simulink model "Simulation_Parallel"  (R2025b)
settings: Solver=ode23tb  StartTime=0.0  StopTime=30000  RelTol=1e-4  AbsTol=1e-4  EnableMultiTasking=on
PreLoadFcn:
  | addpath(genpath(fileparts(bdroot)));
  | disp('Model loaded: Added subfolders to path.');
InitFcn:
  | %if exist('optiver') > 1
  | %    % OptiToolBox is installed
  | %   disp('OptiToolBox is installed');
  | %else
  | %    cd ../OptiToolbox;
  | %    unzip OPTIToolbox.zip;
  |  %   run opti_Install;
  | %    cd ../../../../Loadsharing;
  | % end
  | 
  | clear all
  | %Mpcparam
  | X_init_1;
values from neighbouring files (symbols this model uses):
  X1 = [97725.7043981493 ... (first row only)    [X_init_parallel.m]
  X2 = X1    [X_init_parallel.m]
libraries: simulink x4, slpidlib x3
settings Model: SimulationMode=accelerator  Creator=chancor1  LastModifiedBy=ld719
settings SolverCC: AlgebraicLoopSolver=TrustRegion
settings DataIOCC: LimitDataPoints=on  SaveFinalState=on  SaveFormat=Array  SignalLoggingSaveFormat=ModelDataLogs  ReturnWorkspaceOutputs=off
settings OptimizationCC: ExpressionDepthLimit=2147483647.0  LifeSpan=inf
settings DebuggingCC: UnderspecifiedInitializationDetection=Classic  MergeDetectMultiDrivingBlocksExec=none  SolverPrmCheckMsg=warning  FcnCallInpInsideContextMsg=warning  UnconnectedInputMsg=warning  UnconnectedOutputMsg=warning  UnconnectedLineMsg=warning  StateNameClashWarn=warning  SFUnexpectedBacktrackingDiag=warning  SFNoUnconditionalDefaultTransitionDiag=warning  SFExecutionAtInitializationDiag=none  ArithmeticOperatorsInVariantConditions=warning
settings HardwareCC: ProdBitPerPointer=32.0  ProdBitPerSizeT=32.0  ProdBitPerPtrDiffT=32.0  ProdLargestAtomicFloat=None  ProdIntDivRoundTo=Undefined  ProdEndianess=Unspecified  ProdWordSize=32.0  ProdHWDeviceType=32-bit Generic
settings ModelReferenceCC: EnableRefExpFcnMdlSchedulingChecks=on  PropagateSignalLabelsOutOfModel=off
settings SFSimCC: SimUseLocalCustomCode=off  CustomCodeUndefinedFunction=UseInterfaceOnly
settings RTWCC: RTWUseLocalCustomCode=off  GPUComputeCapability=3.5
settings CodeAppCC: StateflowObjectComments=on
settings GRTTargetCC: TargetLangStandard=C89/C90 (ANSI)  CombineOutputUpdateFcns=off  GRTInterface=on
settings ConfigComp: CovMetricSettings=dw  CovSaveCumulativeToWorkspaceVar=on  CovSaveSingleToWorkspaceVar=on  CovExternalEMLEnable=off  CovSFcnEnable=off

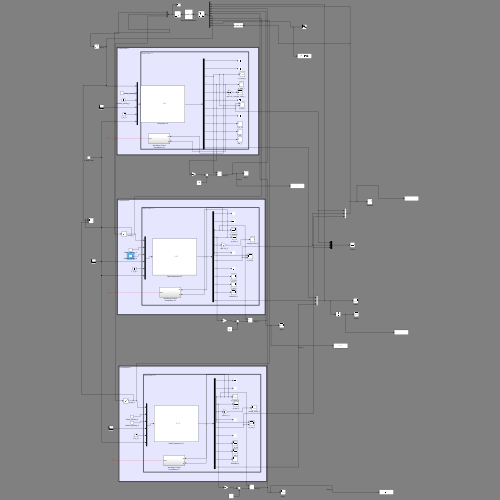
[thumbnail: Simulink's stored preview of the top-level diagram]
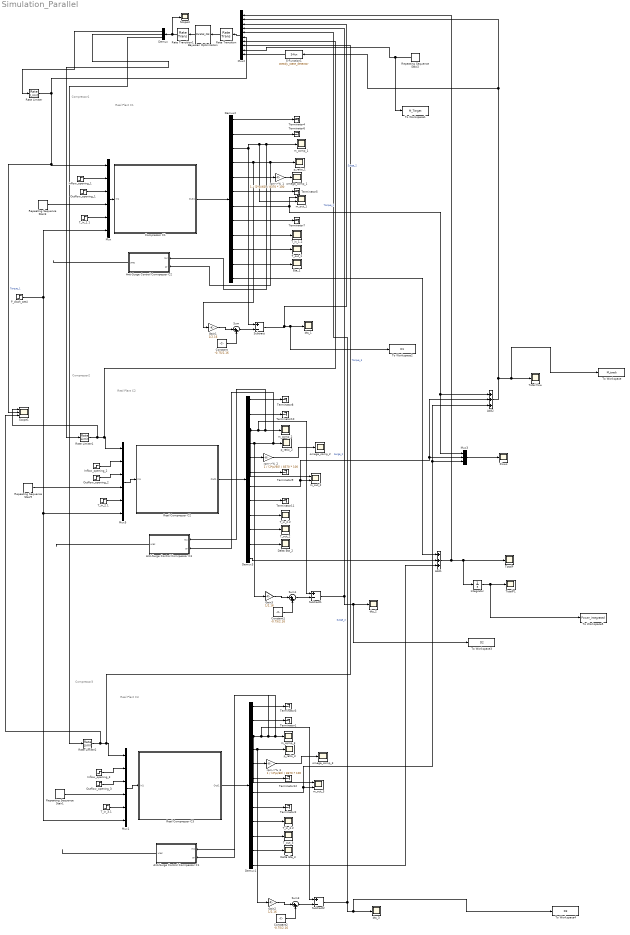
== system Simulation_Parallel ==
  note: Real Plant C2
  note: Real Plant C1
  note: Compressor2
  note: Compressor1
  note: Compressor3
  note: Real Plant C3
  Add1 : Sum  Inputs=+++
  Add2 : Sum  Inputs=+++
  Anti-Surge Control Comrpessor C1 : Subsystem
  Anti-Surge Control Comrpessor C2 : Subsystem
  Anti-Surge Control Comrpessor C3 : Subsystem
  Bayesian Optimization : S-Function  FunctionName=Parallel_CEI  SFunctionDeploymentMode=off  EnableBusSupport=off
  Compressor C1 : Subsystem
      mask Display: image(imread('comp_plant.jpg'))
  Constant : Constant  Value=-0.75/2.16
  Constant1 : Constant  Value=-0.75/2.16
  Constant2 : Constant  Value=-0.75/2.16
  Delta Eta_2 : Scope
      settings: TimeSpan=400  ActiveDisplayYMinimum=0.71048158275738349  ActiveDisplayYMaximum=0.91746637910547824  DataLoggingVariableName=m_rec16  DataLoggingSaveFormat=Array
  Delta Eta_3 : Scope
      settings: TimeSpan=400  ActiveDisplayYMinimum=0.57039067870256488  ActiveDisplayYMaximum=0.76995457969756409  DataLoggingVariableName=m_rec4  DataLoggingSaveFormat=Array
  Demux : Demux  Outputs=3
  Demux1 : Demux  Outputs=12
  Demux2 : Demux  Outputs=12
  Demux3 : Demux  Outputs=12
  Eta_1 : Scope
      settings: TimeSpan=500  ActiveDisplayYMinimum=0.2397543776883454  ActiveDisplayYMaximum=0.63682038343790071  DataLoggingVariableName=m_rec16  DataLoggingSaveFormat=Array
  Flows : Scope
      settings: TimeSpan=500  ActiveDisplayYMinimum=0.36309368835206474  ActiveDisplayYMaximum=0.74236027172168861  DataLoggingVariableName=Individual_Flows  DataLoggingSaveFormat=Array
  Gain1 : Gain  Gain=1/2.16
  Gain2 : Gain  Gain=1/2.16
  Gain3 : Gain  Gain=1/2.16
  Inflow_opening_1 : Step  Time=25  Before=0.4541  After=0.4541  SampleTime=0
  Inflow_opening_2 : Step  Time=25  Before=0.4541  After=0.4541  SampleTime=0
  Inflow_opening_3 : Step  Time=25  Before=0.4541  After=0.4541  SampleTime=0
  Integrator : Integrator
  Mux : Mux  Inputs=6
  Mux1 : Mux  Inputs=6
  Mux2 : Mux  Inputs=10
  Mux3 : Mux  Inputs=3
  Mux5 : Mux  Inputs=6
  Outflow_opening_1 : Step  Time=30  Before=0.56  After=0.56  SampleTime=0
  Outflow_opening_2 : Step  Time=30  Before=0.56  After=0.56  SampleTime=0
  Outflow_opening_3 : Step  Time=30  Before=0.56  After=0.56  SampleTime=0
  P_disch_set4 : Step  Time=4000  Before=155000  After=155000  SampleTime=0
  Rate Limiter : RateLimiter  RisingSlewLimit=0.1  FallingSlewLimit=-0.1  SampleTimeMode=inherited
  Rate Limiter1 : RateLimiter  RisingSlewLimit=0.1  FallingSlewLimit=-0.1  SampleTimeMode=inherited
  Rate Limiter2 : RateLimiter  RisingSlewLimit=0.1  FallingSlewLimit=-0.1  SampleTimeMode=inherited
  Rate Transition : RateTransition
  Rate Transition1 : RateTransition  InitialCondition=[15;15;15]
  Real Compressor C2 : Subsystem
      mask Display: image(imread('comp_plant.jpg'))
  Real Compressor C3 : Subsystem
      mask Display: image(imread('comp_plant.jpg'))
  Repeating Sequence Stair1 : simulink/Sources/Repeating Sequence Stair  OutValues=[0].'  tsamp=-1  OutMin=[]  OutMax=[]  OutDataTypeStr=double  OutputDataTypeScalingMode=double  OutDataType=fixdt(0,8)  ConRadixGroup=Best Precision: Vector-wise  OutScaling=2^-12
  Repeating Sequence Stair2 : simulink/Sources/Repeating Sequence Stair  OutValues=[2.1 1.8 1.9 1.7 1.6 1.5 ].'  tsamp=5000  OutMin=[]  OutMax=[]  OutDataTypeStr=double  OutputDataTypeScalingMode=double  OutDataType=fixdt(0,8)  ConRadixGroup=Best Precision: Vector-wise  OutScaling=2^-12
  Repeating Sequence Stair3 : simulink/Sources/Repeating Sequence Stair  OutValues=[0].'  tsamp=-1  OutMin=[]  OutMax=[]  OutDataTypeStr=double  OutputDataTypeScalingMode=double  OutDataType=fixdt(0,8)  ConRadixGroup=Best Precision: Vector-wise  OutScaling=2^-12
  Repeating Sequence Stair9 : simulink/Sources/Repeating Sequence Stair  OutValues=[0].'  tsamp=-1  OutMin=[]  OutMax=[]  OutDataTypeStr=double  OutputDataTypeScalingMode=double  OutDataType=fixdt(0,8)  ConRadixGroup=Best Precision: Vector-wise  OutScaling=2^-12
  S-Function1 : S-Function  FunctionName=steady_state_detector  SFunctionDeploymentMode=off  EnableBusSupport=off
  Scope1 : Scope  NumInputPorts=3
      settings: ActiveDisplayYMinimum=7.5235070284689751  ActiveDisplayYMaximum=22.497388107947891  DataLoggingVariableName=ScopeData4
  Scope4 : Scope
      settings: ActiveDisplayYMinimum=9.125  ActiveDisplayYMaximum=27.875
  Subtract : Sum  Inputs=+-
  Subtract1 : Sum  Inputs=+-
  Subtract2 : Sum  Inputs=+-
  Sum : Sum  Inputs=|++
  Sum1 : Sum  Inputs=|++
  Sum3 : Sum  Inputs=|++
  T_in_1.1 : Step  Time=2  Before=273+20  After=273+20  SampleTime=0
  T_in_1.2 : Scope
      settings: ActiveDisplayYMinimum=278.35  ActiveDisplayYMaximum=307.65  DataLoggingVariableName=m_rec1  DataLoggingSaveFormat=Array
  T_in_2.1 : Step  Time=2  Before=273+20  After=273+20  SampleTime=0
  T_in_2.2 : Scope
      settings: ActiveDisplayYMinimum=1.41031E-278  ActiveDisplayYMaximum=8E-262  DataLoggingVariableName=m_rec1  DataLoggingSaveFormat=Array
  T_in_3.1 : Step  Time=2  Before=273+20  After=273+20  SampleTime=0
  T_in_3.2 : Scope
      settings: ActiveDisplayYMinimum=1.41031E-278  ActiveDisplayYMaximum=8E-262  DataLoggingVariableName=m_rec5  DataLoggingSaveFormat=Array
  T_out_1 : Scope
      settings: TimeSpan=100  ActiveDisplayYMinimum=335.8022  ActiveDisplayYMaximum=433.80571  DataLoggingVariableName=m_rec2  DataLoggingSaveFormat=Array
  T_out_2 : Scope
      settings: TimeSpan=100  ActiveDisplayYMinimum=370.79785  ActiveDisplayYMaximum=427.9001  DataLoggingVariableName=m_rec2  DataLoggingSaveFormat=Array
  T_out_3 : Scope
      settings: TimeSpan=100  ActiveDisplayYMinimum=370.79785  ActiveDisplayYMaximum=427.9001  DataLoggingVariableName=m_rec6  DataLoggingSaveFormat=Array
  Terminator{1..12} (12 alike) : Terminator
  To Workspace : ToWorkspace  VariableName=M_track  SaveFormat=Structure With Time  SampleTime=1
  To Workspace1 : ToWorkspace  VariableName=M_Target  SaveFormat=Structure With Time  SampleTime=1
  To Workspace2 : ToWorkspace  VariableName=D1  SaveFormat=Structure With Time  SampleTime=1
  To Workspace3 : ToWorkspace  VariableName=D2  SaveFormat=Structure With Time  SampleTime=1
  To Workspace4 : ToWorkspace  VariableName=D3  SaveFormat=Structure With Time  SampleTime=1
  To Workspace5 : ToWorkspace  VariableName=Power_integrated  SaveFormat=Structure With Time  SampleTime=1
  Total flow : Scope
      settings: TimeSpan=30000  ActiveDisplayYMinimum=1.2722600118252789  ActiveDisplayYMaximum=2.1997897754564577  DataLoggingVariableName=Individual_Flows1  DataLoggingSaveFormat=Array
  TotalP : Scope
      settings: ActiveDisplayYMinimum=126510.3736500807  ActiveDisplayYMaximum=352840.8765047628  DataLoggingVariableName=TotalP  DataLoggingSaveFormat=Array
  TotalP1 : Scope
      settings: ActiveDisplayYMinimum=6.1318455800186586E+9  ActiveDisplayYMaximum=6.1318558553426237E+9  DataLoggingVariableName=TotalE  DataLoggingSaveFormat=Array
  dts_1 : Scope
      settings: TimeSpan=500  ActiveDisplayYMinimum=0.005652196127564145  ActiveDisplayYMaximum=0.23223162651311186  DataLoggingVariableName=m_rec  DataLoggingSaveFormat=Array
  dts_2 : Scope
      settings: TimeSpan=500  ActiveDisplayYMinimum=-0.014136511221945931  ActiveDisplayYMaximum=0.23443037177416717  DataLoggingVariableName=m_rec3  DataLoggingSaveFormat=Array
  dts_3 : Scope
      settings: TimeSpan=500  ActiveDisplayYMinimum=-0.030750707158997012  ActiveDisplayYMaximum=0.23627639354495333  DataLoggingVariableName=m_rec7  DataLoggingSaveFormat=Array
  m_comp_1 : Scope
      settings: TimeSpan=100  ActiveDisplayYMinimum=60.15587  ActiveDisplayYMaximum=126.64848  DataLoggingVariableName=m_comp_C1  DataLoggingSaveFormat=Array
  m_comp_2 : Scope
      settings: TimeSpan=100  ActiveDisplayYMinimum=38.57766  ActiveDisplayYMaximum=113.2372  DataLoggingVariableName=m_comp_C2  DataLoggingSaveFormat=Array
  m_comp_3 : Scope
      settings: TimeSpan=100  ActiveDisplayYMinimum=38.57766  ActiveDisplayYMaximum=113.2372  DataLoggingVariableName=m_comp_C  DataLoggingSaveFormat=Array
  m_out_1 : Scope  NumInputPorts=2
      settings: ActiveDisplayYMinimum=0.47698487803056794  ActiveDisplayYMaximum=0.61709914190973469  DataLoggingVariableName=ScopeData3
  m_out_2 : Scope  NumInputPorts=2
      settings: ActiveDisplayYMinimum=61.12166  ActiveDisplayYMaximum=116.4647  DataLoggingVariableName=ScopeData2
  m_out_3 : Scope  NumInputPorts=2
      settings: ActiveDisplayYMinimum=-1  ActiveDisplayYMaximum=1
  omega_comp_1 : Scope
      settings: TimeSpan=10  ActiveDisplayYMinimum=55.77307  ActiveDisplayYMaximum=77.75846  DataLoggingVariableName=ScopeData5
  omega_comp_2 : Scope
      settings: TimeSpan=10  ActiveDisplayYMinimum=20000  ActiveDisplayYMaximum=120000  DataLoggingVariableName=ScopeData5
  omega_comp_3 : Scope
      settings: TimeSpan=10  ActiveDisplayYMinimum=20000  ActiveDisplayYMaximum=120000  DataLoggingVariableName=ScopeData6
  p_ratio_1 : Scope
      settings: TimeSpan=20  ActiveDisplayYMinimum=1.533809798369548  ActiveDisplayYMaximum=1.8504440162741049  DataLoggingVariableName=p_ratio_C1  DataLoggingSaveFormat=Array
  p_ratio_2 : Scope
      settings: TimeSpan=20  ActiveDisplayYMinimum=-1  ActiveDisplayYMaximum=1  DataLoggingVariableName=p_ratio_C2  DataLoggingSaveFormat=Array
  p_ratio_3 : Scope
      settings: TimeSpan=20  ActiveDisplayYMinimum=-1  ActiveDisplayYMaximum=1  DataLoggingVariableName=p_ratio_C  DataLoggingSaveFormat=Array
  rpm->%_1 : Gain  Gain=1 / (2*pi/60) / 8370 * 100
  rpm->%_2 : Gain  Gain=1 / (2*pi/60) / 8370 * 100
  rpm->%_3 : Gain  Gain=1 / (2*pi/60) / 8370 * 100
  wires:
  Demux2/7 -> m_out_1/1, Mux3/1, Add2/1
  Demux3/7 -> Add2/2, Mux3/2, m_out_2/2
  Mux3/1 -> Flows/1
  Demux3/12 -> Add1/2
  Demux2/12 -> Add1/1
  Demux2/11 -> Eta_1/1
  Demux2/4 -> Gain1/1, Anti-Surge Control Comrpessor C2/2(pr), p_ratio_1/1
  Demux2/3 -> Anti-Surge Control Comrpessor C2/1(mc), m_comp_1/1, m_out_1/2, Subtract/1
  T_in_1.1/1 -> Mux/5
  Outflow_opening_1/1 -> Mux/3
  Inflow_opening_1/1 -> Mux/2
  Demux3/11 -> Delta Eta_2/1
  Demux3/4 -> Anti-Surge Control Comrpessor C3/2(pr), p_ratio_2/1, Gain3/1
  Demux3/3 -> Subtract1/1, Anti-Surge Control Comrpessor C3/1(mc), m_comp_2/1, m_out_2/1
  T_in_2.1/1 -> Mux5/5
  Outflow_opening_2/1 -> Mux5/3
  Inflow_opening_2/1 -> Mux5/2
  P_disch_set4/1 -> Mux1/6, Mux5/6, Mux/6
  Compressor C1/1(Out1) -> Demux2/1
  Mux/1 -> Compressor C1/1(In1)
  rpm->%_1/1 -> omega_comp_1/1
  Demux2/10 -> T_out_1/1
  Demux2/9 -> T_in_1.2/1
  Demux2/8 -> Terminator7/1
  Demux2/2 -> Terminator6/1
  Demux2/1 -> Terminator4/1
  Demux2/6 -> Terminator5/1
  Demux2/5 -> rpm->%_1/1
  Real Compressor C2/1(Out1) -> Demux3/1
  Mux5/1 -> Real Compressor C2/1(In1)
  rpm->%_2/1 -> omega_comp_2/1
  Demux3/10 -> T_out_2/1
  Demux3/9 -> T_in_2.2/1
  Demux3/8 -> Terminator11/1
  Demux3/2 -> Terminator10/1
  Demux3/1 -> Terminator8/1
  Demux3/6 -> Terminator9/1
  Demux3/5 -> rpm->%_2/1
  Sum/1 -> Subtract/2
  Gain1/1 -> Sum/1
  Constant/1 -> Sum/2
  Gain3/1 -> Sum1/1
  Constant1/1 -> Sum1/2
  Sum1/1 -> Subtract1/2
  Rate Transition1/1 -> Scope4/1, Demux/1
  Rate Transition/1 -> Bayesian Optimization/1
  Mux2/1 -> Rate Transition/1
  Bayesian Optimization/1 -> Rate Transition1/1
  Add1/1 -> TotalP/1, Integrator/1, Mux2/1
  Demux/1 -> Rate Limiter/1
  Rate Limiter/1 -> Mux2/6, Scope1/2, Mux/1  "Torque_1"
  Demux/2 -> Rate Limiter1/1
  Rate Limiter1/1 -> Scope1/1, Mux2/7, Mux5/1  "Torque_2"
  S-Function1/1 -> Mux2/10
  Constant2/1 -> Sum3/2
  Demux1/3 -> Subtract2/1, Anti-Surge Control Comrpessor C1/1(mc), Anti-Surge Control Comrpessor C1/2(pr), m_comp_3/1, m_out_3/1
  T_in_3.1/1 -> Mux1/5
  Demux/3 -> Rate Limiter2/1
  rpm->%_3/1 -> omega_comp_3/1
  Demux1/6 -> Terminator12/1
  Outflow_opening_3/1 -> Mux1/3
  Real Compressor C3/1(Out1) -> Demux1/1
  Gain2/1 -> Sum3/1
  Sum3/1 -> Subtract2/2
  Demux1/7 -> Add2/3, Mux3/3, m_out_3/2
  Demux1/9 -> T_in_3.2/1
  Mux1/1 -> Real Compressor C3/1(In1)
  Demux1/8 -> Terminator2/1
  Rate Limiter2/1 -> Scope1/3, Mux2/8, Mux1/1  "Torque_3"
  Demux1/10 -> T_out_3/1
  Demux1/4 -> p_ratio_3/1, Gain2/1
  Demux1/1 -> Terminator3/1
  Inflow_opening_3/1 -> Mux1/2
  Demux1/11 -> Delta Eta_3/1
  Demux1/5 -> rpm->%_3/1
  Demux1/12 -> Add1/3
  Demux1/2 -> Terminator1/1
  Repeating Sequence Stair2/1 -> Mux2/9, To Workspace1/1
  Add2/1 -> S-Function1/1, Mux2/2, To Workspace/1, Total flow/1
  Subtract/1 -> Mux2/3, To Workspace2/1, dts_1/1  "Surge_2"
  Subtract1/1 -> Mux2/4, To Workspace3/1, dts_2/1  "Surge_2"
  Subtract2/1 -> Mux2/5, To Workspace4/1, dts_3/1  "Surge_2"
  Integrator/1 -> To Workspace5/1, TotalP1/1
  Anti-Surge Control Comrpessor C2/1(urec) -> ?
  Anti-Surge Control Comrpessor C3/1(urec) -> ?
  Anti-Surge Control Comrpessor C1/1(urec) -> ?
  Repeating Sequence Stair3/1 -> Mux/4
  Repeating Sequence Stair9/1 -> Mux5/4
  Repeating Sequence Stair1/1 -> Mux1/4

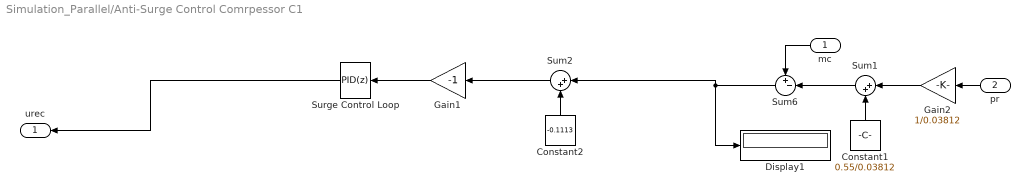
== system Simulation_Parallel/Anti-Surge Control Comrpessor C1 ==
  mc : Inport
  pr : Inport  Port=2
  Constant1 : Constant  Value=0.55/0.03812
  Constant2 : Constant  Value=-0.1113
  Display1 : Display
  Gain1 : Gain  Gain=-1
  Gain2 : Gain  Gain=1/0.03812
  Sum1 : Sum  Inputs=|++
  Sum2 : Sum  Inputs=|++
  Sum6 : Sum  Inputs=+-|
  Surge Control Loop : slpidlib/PID Controller  Controller=PID  Form=Parallel  TimeDomain=Discrete-time  UseExternalTs=off  SampleTime=0.5  IntegratorMethod=Forward Euler  FilterMethod=Forward Euler  ControllerParametersSource=internal  P=0.05  I=0.01  UseKiTs=off  D=0  UseExternalDerivativeSource=off  N=2.82959055969234  UseFilter=on  TunerSelectOption=Transfer Function Based (PID Tuner App)  ZeroCross=off  InitialConditionSource=internal  InitialConditionForIntegrator=0  InitialConditionForFilter=0  DifferentiatorICPrevScaledInput=0  ExternalReset=none  TrackingMode=off  Kt=1  LimitOutput=on  SatLimitsSource=internal  UpperSaturationLimit=1  LowerSaturationLimit=0  LinearizeAsGain=off  AntiWindupMode=back-calculation  Kb=1  LimitIntegrator=off  UpperIntegratorSaturationLimit=inf  LowerIntegratorSaturationLimit=-inf  POutMin=[]  POutMax=[]  IOutMin=[]  IOutMax=[]  DOutMin=[]  DOutMax=[]  NOutMin=[]  NOutMax=[]  SumOutMin=[]  SumOutMax=[]  SaturationOutMin=[]  SaturationOutMax=[]  PParamMin=[]  PParamMax=[]  IParamMin=[]  IParamMax=[]  DParamMin=[]  DParamMax=[]  NParamMin=[]  NParamMax=[]  KbParamMin=[]  KbParamMax=[]  KtParamMin=[]  KtParamMax=[]  KbOutMin=[]  KbOutMax=[]  KtOutMin=[]  KtOutMax=[]  IntegratorOutMin=[]  IntegratorOutMax=[]  FilterOutMin=[]  FilterOutMax=[]  SumI1OutMin=[]  SumI1OutMax=[]  SumI2OutMin=[]  SumI2OutMax=[]  SumI3OutMin=[]  SumI3OutMax=[]  SumI4OutMin=[]  SumI4OutMax=[]  SumDOutMin=[]  SumDOutMax=[]  DifferentiatorOutMin=[]  DifferentiatorOutMax=[]  FilterDiffOutCoefMin=[]  FilterDiffOutCoefMax=[]  ReciprocalOutMin=[]  ReciprocalOutMax=[]  SumDenOutMin=[]  SumDenOutMax=[]  SumNumOutMin=[]  SumNumOutMax=[]  DivideOutMin=[]  DivideOutMax=[]  UdiffTsProdOutMin=[]  UdiffTsProdOutMax=[]  NTsProdOutMin=[]  NTsProdOutMax=[]  UintegralTsProdOutMin=[]  UintegralTsProdOutMax=[]  UngainTsProdOutMin=[]  UngainTsProdOutMax=[]  ClampingZeroOutDataTypeStr=Inherit: Inherit via back propagation  ClampingZeroOutMin=[]  ClampingZeroOutMax=[]  FilterDenConstantOutDataTypeStr=Inherit: Inherit via back propagation  FilterDenConstantOutMin=[]  FilterDenConstantOutMax=[]  PCopyOutDataTypeStr=Inherit: Inherit via back propagation  PCopyOutMin=[]  PCopyOutMax=[]  NCopyOutDataTypeStr=Inherit: Inherit via back propagation  NCopyOutMin=[]  NCopyOutMax=[]  IntegratorContinuousStateAttributes=''  IntegratorStateMustResolveToSignalObject=off  IntegratorRTWStateStorageClass=Auto  FilterContinuousStateAttributes=''  FilterStateMustResolveToSignalObject=off  FilterRTWStateStorageClass=Auto  ParallelPVariant=InternalParameters  IdealPVariant=Disabled  IVariant=InternalParameters  DVariant=InternalParameters  IntegratorVariant=Discrete  SatVariant=Enabled  AWVariant=BackCalculation  PCopyVariant=Disabled  TRVariant=Disabled  FdbkBlocksVariant=Forward  IdealPFdbkVariant=Disabled  SatFdbkVariant=Disabled  DerivativeFilterVariant=ForwardEulerFilter  NVariant=InternalParameters  NCopyVariant=Disabled  FilterICVariant=InternalICsFilter  IntegratorICVariant=InternalICs  ExternalResetVariant=Disabled  TRSumVariant=Passthrough  SumFdbkVariant=Disabled  SumVariant=Sum_PID  TsampFilterVariant=InternalTs  TsampNgainVariant=Passthrough  TsampIntegralVariant=Disabled_SignalSpec  ExternalSaturationOutDataTypeStr=Inherit: Same as second input  DerivativeSourceVariant=ErrorSignal  PreIntVariant=InternalPreInt
  urec : Outport
  wires:
  Gain2/1 -> Sum1/1
  Constant1/1 -> Sum1/2
  Sum1/1 -> Sum6/2
  Sum6/1 -> Sum2/1, Display1/1
  Surge Control Loop/1 -> urec/1
  mc/1 -> Sum6/1
  pr/1 -> Gain2/1
  Gain1/1 -> Surge Control Loop/1
  Sum2/1 -> Gain1/1
  Constant2/1 -> Sum2/2

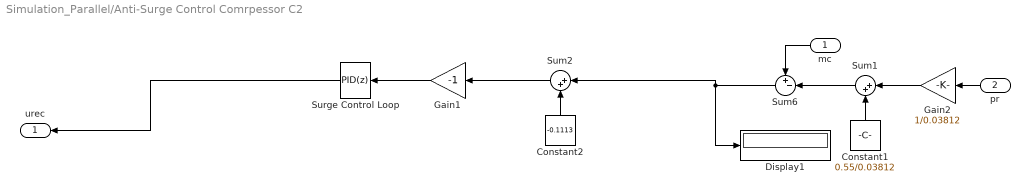
== system Simulation_Parallel/Anti-Surge Control Comrpessor C2 ==
  mc : Inport
  pr : Inport  Port=2
  Constant1 : Constant  Value=0.55/0.03812
  Constant2 : Constant  Value=-0.1113
  Display1 : Display
  Gain1 : Gain  Gain=-1
  Gain2 : Gain  Gain=1/0.03812
  Sum1 : Sum  Inputs=|++
  Sum2 : Sum  Inputs=|++
  Sum6 : Sum  Inputs=+-|
  Surge Control Loop : slpidlib/PID Controller  Controller=PID  Form=Parallel  TimeDomain=Discrete-time  UseExternalTs=off  SampleTime=0.5  IntegratorMethod=Forward Euler  FilterMethod=Forward Euler  ControllerParametersSource=internal  P=0.05  I=0.01  UseKiTs=off  D=0  UseExternalDerivativeSource=off  N=2.82959055969234  UseFilter=on  TunerSelectOption=Transfer Function Based (PID Tuner App)  ZeroCross=off  InitialConditionSource=internal  InitialConditionForIntegrator=0  InitialConditionForFilter=0  DifferentiatorICPrevScaledInput=0  ExternalReset=none  TrackingMode=off  Kt=1  LimitOutput=on  SatLimitsSource=internal  UpperSaturationLimit=1  LowerSaturationLimit=0  LinearizeAsGain=off  AntiWindupMode=back-calculation  Kb=1  LimitIntegrator=off  UpperIntegratorSaturationLimit=inf  LowerIntegratorSaturationLimit=-inf  POutMin=[]  POutMax=[]  IOutMin=[]  IOutMax=[]  DOutMin=[]  DOutMax=[]  NOutMin=[]  NOutMax=[]  SumOutMin=[]  SumOutMax=[]  SaturationOutMin=[]  SaturationOutMax=[]  PParamMin=[]  PParamMax=[]  IParamMin=[]  IParamMax=[]  DParamMin=[]  DParamMax=[]  NParamMin=[]  NParamMax=[]  KbParamMin=[]  KbParamMax=[]  KtParamMin=[]  KtParamMax=[]  KbOutMin=[]  KbOutMax=[]  KtOutMin=[]  KtOutMax=[]  IntegratorOutMin=[]  IntegratorOutMax=[]  FilterOutMin=[]  FilterOutMax=[]  SumI1OutMin=[]  SumI1OutMax=[]  SumI2OutMin=[]  SumI2OutMax=[]  SumI3OutMin=[]  SumI3OutMax=[]  SumI4OutMin=[]  SumI4OutMax=[]  SumDOutMin=[]  SumDOutMax=[]  DifferentiatorOutMin=[]  DifferentiatorOutMax=[]  FilterDiffOutCoefMin=[]  FilterDiffOutCoefMax=[]  ReciprocalOutMin=[]  ReciprocalOutMax=[]  SumDenOutMin=[]  SumDenOutMax=[]  SumNumOutMin=[]  SumNumOutMax=[]  DivideOutMin=[]  DivideOutMax=[]  UdiffTsProdOutMin=[]  UdiffTsProdOutMax=[]  NTsProdOutMin=[]  NTsProdOutMax=[]  UintegralTsProdOutMin=[]  UintegralTsProdOutMax=[]  UngainTsProdOutMin=[]  UngainTsProdOutMax=[]  ClampingZeroOutDataTypeStr=Inherit: Inherit via back propagation  ClampingZeroOutMin=[]  ClampingZeroOutMax=[]  FilterDenConstantOutDataTypeStr=Inherit: Inherit via back propagation  FilterDenConstantOutMin=[]  FilterDenConstantOutMax=[]  PCopyOutDataTypeStr=Inherit: Inherit via back propagation  PCopyOutMin=[]  PCopyOutMax=[]  NCopyOutDataTypeStr=Inherit: Inherit via back propagation  NCopyOutMin=[]  NCopyOutMax=[]  IntegratorContinuousStateAttributes=''  IntegratorStateMustResolveToSignalObject=off  IntegratorRTWStateStorageClass=Auto  FilterContinuousStateAttributes=''  FilterStateMustResolveToSignalObject=off  FilterRTWStateStorageClass=Auto  ParallelPVariant=InternalParameters  IdealPVariant=Disabled  IVariant=InternalParameters  DVariant=InternalParameters  IntegratorVariant=Discrete  SatVariant=Enabled  AWVariant=BackCalculation  PCopyVariant=Disabled  TRVariant=Disabled  FdbkBlocksVariant=Forward  IdealPFdbkVariant=Disabled  SatFdbkVariant=Disabled  DerivativeFilterVariant=ForwardEulerFilter  NVariant=InternalParameters  NCopyVariant=Disabled  FilterICVariant=InternalICsFilter  IntegratorICVariant=InternalICs  ExternalResetVariant=Disabled  TRSumVariant=Passthrough  SumFdbkVariant=Disabled  SumVariant=Sum_PID  TsampFilterVariant=InternalTs  TsampNgainVariant=Passthrough  TsampIntegralVariant=Disabled_SignalSpec  ExternalSaturationOutDataTypeStr=Inherit: Same as second input  DerivativeSourceVariant=ErrorSignal  PreIntVariant=InternalPreInt
  urec : Outport
  wires:
  Gain2/1 -> Sum1/1
  Constant1/1 -> Sum1/2
  Sum1/1 -> Sum6/2
  Sum6/1 -> Sum2/1, Display1/1
  Surge Control Loop/1 -> urec/1
  mc/1 -> Sum6/1
  pr/1 -> Gain2/1
  Gain1/1 -> Surge Control Loop/1
  Sum2/1 -> Gain1/1
  Constant2/1 -> Sum2/2

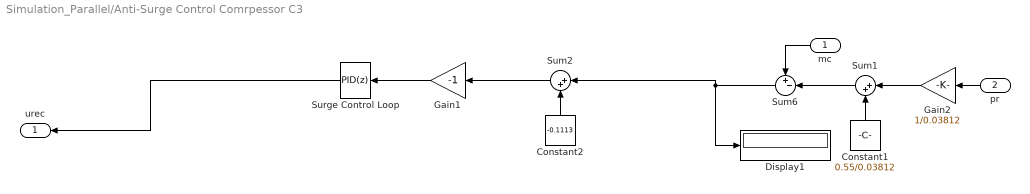
== system Simulation_Parallel/Anti-Surge Control Comrpessor C3 ==
  mc : Inport
  pr : Inport  Port=2
  Constant1 : Constant  Value=0.55/0.03812
  Constant2 : Constant  Value=-0.1113
  Display1 : Display
  Gain1 : Gain  Gain=-1
  Gain2 : Gain  Gain=1/0.03812
  Sum1 : Sum  Inputs=|++
  Sum2 : Sum  Inputs=|++
  Sum6 : Sum  Inputs=+-|
  Surge Control Loop : slpidlib/PID Controller  Controller=PID  Form=Parallel  TimeDomain=Discrete-time  UseExternalTs=off  SampleTime=0.5  IntegratorMethod=Forward Euler  FilterMethod=Forward Euler  ControllerParametersSource=internal  P=0.05  I=0.01  UseKiTs=off  D=0  UseExternalDerivativeSource=off  N=2.82959055969234  UseFilter=on  TunerSelectOption=Transfer Function Based (PID Tuner App)  ZeroCross=off  InitialConditionSource=internal  InitialConditionForIntegrator=0  InitialConditionForFilter=0  DifferentiatorICPrevScaledInput=0  ExternalReset=none  TrackingMode=off  Kt=1  LimitOutput=on  SatLimitsSource=internal  UpperSaturationLimit=1  LowerSaturationLimit=0  LinearizeAsGain=off  AntiWindupMode=back-calculation  Kb=1  LimitIntegrator=off  UpperIntegratorSaturationLimit=inf  LowerIntegratorSaturationLimit=-inf  POutMin=[]  POutMax=[]  IOutMin=[]  IOutMax=[]  DOutMin=[]  DOutMax=[]  NOutMin=[]  NOutMax=[]  SumOutMin=[]  SumOutMax=[]  SaturationOutMin=[]  SaturationOutMax=[]  PParamMin=[]  PParamMax=[]  IParamMin=[]  IParamMax=[]  DParamMin=[]  DParamMax=[]  NParamMin=[]  NParamMax=[]  KbParamMin=[]  KbParamMax=[]  KtParamMin=[]  KtParamMax=[]  KbOutMin=[]  KbOutMax=[]  KtOutMin=[]  KtOutMax=[]  IntegratorOutMin=[]  IntegratorOutMax=[]  FilterOutMin=[]  FilterOutMax=[]  SumI1OutMin=[]  SumI1OutMax=[]  SumI2OutMin=[]  SumI2OutMax=[]  SumI3OutMin=[]  SumI3OutMax=[]  SumI4OutMin=[]  SumI4OutMax=[]  SumDOutMin=[]  SumDOutMax=[]  DifferentiatorOutMin=[]  DifferentiatorOutMax=[]  FilterDiffOutCoefMin=[]  FilterDiffOutCoefMax=[]  ReciprocalOutMin=[]  ReciprocalOutMax=[]  SumDenOutMin=[]  SumDenOutMax=[]  SumNumOutMin=[]  SumNumOutMax=[]  DivideOutMin=[]  DivideOutMax=[]  UdiffTsProdOutMin=[]  UdiffTsProdOutMax=[]  NTsProdOutMin=[]  NTsProdOutMax=[]  UintegralTsProdOutMin=[]  UintegralTsProdOutMax=[]  UngainTsProdOutMin=[]  UngainTsProdOutMax=[]  ClampingZeroOutDataTypeStr=Inherit: Inherit via back propagation  ClampingZeroOutMin=[]  ClampingZeroOutMax=[]  FilterDenConstantOutDataTypeStr=Inherit: Inherit via back propagation  FilterDenConstantOutMin=[]  FilterDenConstantOutMax=[]  PCopyOutDataTypeStr=Inherit: Inherit via back propagation  PCopyOutMin=[]  PCopyOutMax=[]  NCopyOutDataTypeStr=Inherit: Inherit via back propagation  NCopyOutMin=[]  NCopyOutMax=[]  IntegratorContinuousStateAttributes=''  IntegratorStateMustResolveToSignalObject=off  IntegratorRTWStateStorageClass=Auto  FilterContinuousStateAttributes=''  FilterStateMustResolveToSignalObject=off  FilterRTWStateStorageClass=Auto  ParallelPVariant=InternalParameters  IdealPVariant=Disabled  IVariant=InternalParameters  DVariant=InternalParameters  IntegratorVariant=Discrete  SatVariant=Enabled  AWVariant=BackCalculation  PCopyVariant=Disabled  TRVariant=Disabled  FdbkBlocksVariant=Forward  IdealPFdbkVariant=Disabled  SatFdbkVariant=Disabled  DerivativeFilterVariant=ForwardEulerFilter  NVariant=InternalParameters  NCopyVariant=Disabled  FilterICVariant=InternalICsFilter  IntegratorICVariant=InternalICs  ExternalResetVariant=Disabled  TRSumVariant=Passthrough  SumFdbkVariant=Disabled  SumVariant=Sum_PID  TsampFilterVariant=InternalTs  TsampNgainVariant=Passthrough  TsampIntegralVariant=Disabled_SignalSpec  ExternalSaturationOutDataTypeStr=Inherit: Same as second input  DerivativeSourceVariant=ErrorSignal  PreIntVariant=InternalPreInt
  urec : Outport
  wires:
  Gain2/1 -> Sum1/1
  Constant1/1 -> Sum1/2
  Sum1/1 -> Sum6/2
  Sum6/1 -> Sum2/1, Display1/1
  Surge Control Loop/1 -> urec/1
  mc/1 -> Sum6/1
  pr/1 -> Gain2/1
  Gain1/1 -> Surge Control Loop/1
  Sum2/1 -> Gain1/1
  Constant2/1 -> Sum2/2

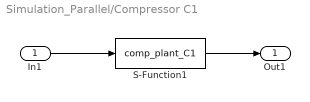
== system Simulation_Parallel/Compressor C1 ==
  In1 : Inport
  S-Function1 : S-Function  FunctionName=comp_plant_C1  Parameters=[], X1  SFunctionDeploymentMode=off  EnableBusSupport=off
  Out1 : Outport
  wires:
  S-Function1/1 -> Out1/1
  In1/1 -> S-Function1/1

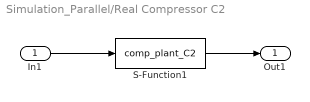
== system Simulation_Parallel/Real Compressor C2 ==
  In1 : Inport
  S-Function1 : S-Function  FunctionName=comp_plant_C2  Parameters=[], X2  SFunctionDeploymentMode=off  EnableBusSupport=off
  Out1 : Outport
  wires:
  S-Function1/1 -> Out1/1
  In1/1 -> S-Function1/1

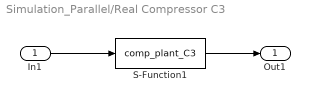
== system Simulation_Parallel/Real Compressor C3 ==
  In1 : Inport
  S-Function1 : S-Function  FunctionName=comp_plant_C3  Parameters=[], X2  SFunctionDeploymentMode=off  EnableBusSupport=off
  Out1 : Outport
  wires:
  S-Function1/1 -> Out1/1
  In1/1 -> S-Function1/1
